simulink model "Dual_Electric_Plant"  (R2021a)
settings: Solver=VariableStepAuto  StartTime=0.0  StopTime=60  RelTol=1e-3  AbsTol=1e-3
InitFcn:
  | Model_Parameters;
undefined symbols (not defined in the file or in its folder): Battery, Electric_Motor, Fuel_Cell
libraries: fl_lib x18, ee_lib x9, nesl_utility x6
settings Model: Creator=jsagardu  LastModifiedBy=LENOVO
settings SolverCC: AutoScaleAbsTol=off  AlgebraicLoopSolver=TrustRegion
settings DebuggingCC: SymbolicDimsDataTypeCodeGenerationDiagnostic=none  SFMachineParentedDataDiag=warning
settings SFSimCC: CustomCodeUndefinedFunction=UseInterfaceOnly
settings SimscapeCC: SimscapeLogType=local  SimscapeLogOpenViewer=on  SimscapeLogLimitData=off  SimscapeLogDataHistory=10000

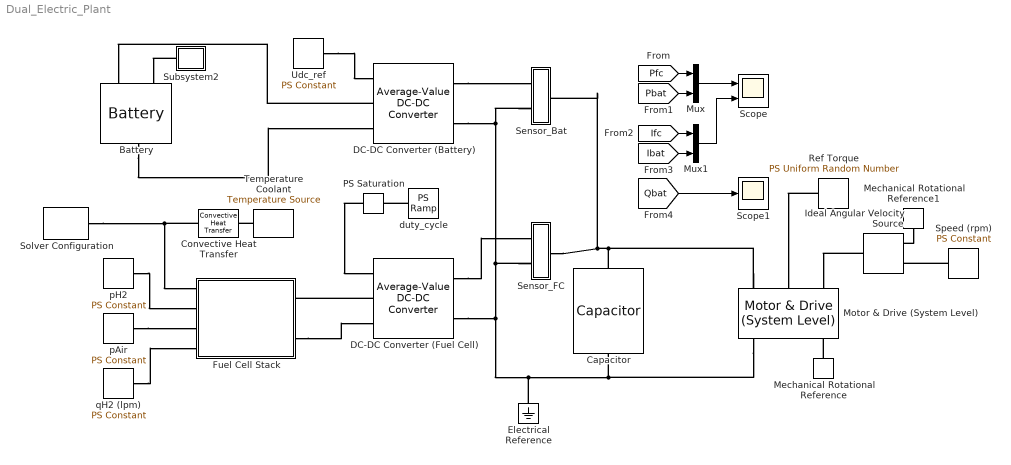
== system Dual_Electric_Plant ==
  Battery : ee_lib/Sources/Battery  Vnom=Battery.Unom V  prm_dir=1  R1_dis=2 Ohm  R1_ch=2 Ohm  R1=Battery.Resistance Ohm  prm_AH=2  AH=Battery.Qnom hr*A  V1=Battery.U1 V  AH1=Battery.Q1 hr*A  prm_R2=1  R2=2000 Ohm  prm_dyn=1  Rp1=0.005 Ohm  tau1=30 s  Rp2=0.005 Ohm  tau2=30 s  Rp3=0.005 Ohm  tau3=30 s  Rp4=0.005 Ohm  tau4=30 s  Rp5=0.005 Ohm  tau5=30 s  prm_fade=1  N_fade=100  AH_fade=45 hr*A  R1_fade=2.02 Ohm  R1_ch_fade=2.02 Ohm  V1_fade=10.35 V  prm_age=1  prm_age_OCV=1  OCV_age=0.9  SOC_age=60  Tmeas_age=298.15 K  delta_time_age_vec=[0] d  temperature_age_vec=[273] K  OCV_scaling_age=2.2134e6  OCV_offset_age=1.632e6  temp_exp_age=0.515833569 V  t_exp_age=0.75  i_specify=off  i_priority=None  i=0 A  i_nominal_specify=off  i_nominal_unit=A  i_nominal_value=1  v_specify=on  v_priority=High  v=Battery.Uinit V  v_nominal_specify=off  v_nominal_unit=V  v_nominal_value=1  charge_specify=on  charge_priority=High  charge=Battery.Qnom hr*A  charge_nominal_specify=off  charge_nominal_unit=hr*A  charge_nominal_value=1  num_cycles_specify=off  num_cycles_priority=High  num_cycles=0  num_cycles_nominal_specify=off  num_cycles_nominal_unit=1  num_cycles_nominal_value=1  thermal_mass=30000 J/K  Tmeas=298.15 K  Vnom_T2=12 V  R1_T2=2.2 Ohm  R1_T2_dis=2.2 Ohm  R1_T2_ch=2.2 Ohm  V1_T2=11.4 V  R2_T2=2200 Ohm  Rp1_T2=0.005 Ohm  tau1_T2=30 s  Rp2_T2=0.005 Ohm  tau2_T2=30 s  Rp3_T2=0.005 Ohm  tau3_T2=30 s  Rp4_T2=0.005 Ohm  tau4_T2=30 s  Rp5_T2=0.005 Ohm  tau5_T2=30 s  Tmeas2=273.15 K  temperature_specify=off  temperature_priority=High  temperature=298.15 K  temperature_nominal_specify=off  temperature_nominal_unit=K  temperature_nominal_value=1
      settings: LogSimulationData=on  InternalSimscapePortConfiguration="{\"Bottom\":[],\"Left\":[{\"id\":\"p\",\"label\":\"+\",\"type\":\"foundation.electrical.electrical\"},{\"id\":\"q\",\"label\":\"q\",\"type\":\"output\"}],\"Right\":[{\"id\":\"n\",\"label\":\"-\",\"type\":\"foundation.electrical.electrical\"}],\"Top\":[]}"
  Capacitor : fl_lib/Electrical/Electrical Elements/Capacitor  c=5 mF  r=0.05 Ohm  g=0 1/Ohm  i_specify=off  i_priority=None  i=0 A  i_nominal_specify=off  i_nominal_unit=A  i_nominal_value=1  v_specify=off  v_priority=None  v=0 V  v_nominal_specify=off  v_nominal_unit=V  v_nominal_value=1  vc_specify=on  vc_priority=High  vc=500 V  vc_nominal_specify=off  vc_nominal_unit=V  vc_nominal_value=1
  Convective Heat Transfer : fl_lib/Thermal/Thermal Elements/Convective Heat Transfer  area=300 cm^2  heat_tr_coeff=75 W/(m^2 * K)  T_specify=off  T_priority=None  T=0 K  T_nominal_specify=off  T_nominal_unit=K  T_nominal_value=1  Q_specify=off  Q_priority=None  Q=0 W  Q_nominal_specify=off  Q_nominal_unit=W  Q_nominal_value=1
  DC-DC Converter (Battery) : ee_lib/Semiconductors & Converters/Converters/Average-Value DC-DC Converter  control_option=ee.enum.converters.controlinput.voltage  converter_type=ee.enum.converters.dcdctype.boost  efficiency_option=ee.enum.converters.efficiency.constant  efficiency_fixed=100  i_vec=[0, 2, 5] A  efficiency_vec=[90, 95, 98]
      settings: SourceProductBaseCode=PS  LogSimulationData=on  InternalSimscapePortConfiguration="{\"Bottom\":[],\"Left\":[{\"id\":\"Vref\",\"label\":\"Vref\",\"type\":\"input\"},{\"id\":\"p1\",\"label\":\"1+\",\"type\":\"foundation.electrical.electrical\"},{\"id\":\"n1\",\"label\":\"1-\",\"type\":\"foundation.electrical.electrical\"}],\"Right\":[{\"id\":\"p2\",\"label\":\"2+\",\"type\":\"foundation.electrical.electrical\"},{\"id\":\"n2\",\"label\":\"2-\",\"type\":\"foundation.electrical.electrical\"}],\"Top\":[]}"
  DC-DC Converter (Fuel Cell) : ee_lib/Semiconductors & Converters/Converters/Average-Value DC-DC Converter  control_option=ee.enum.converters.controlinput.dutycycle  converter_type=ee.enum.converters.dcdctype.boost  efficiency_option=ee.enum.converters.efficiency.constant  efficiency_fixed=100  i_vec=[0, 2, 5] A  efficiency_vec=[90, 95, 98]
      settings: SourceProductBaseCode=PS  LogSimulationData=on  InternalSimscapePortConfiguration="{\"Bottom\":[],\"Left\":[{\"id\":\"DutyCycle\",\"label\":\"DutyCycle\",\"type\":\"input\"},{\"id\":\"p1\",\"label\":\"1+\",\"type\":\"foundation.electrical.electrical\"},{\"id\":\"n1\",\"label\":\"1-\",\"type\":\"foundation.electrical.electrical\"}],\"Right\":[{\"id\":\"p2\",\"label\":\"2+\",\"type\":\"foundation.electrical.electrical\"},{\"id\":\"n2\",\"label\":\"2-\",\"type\":\"foundation.electrical.electrical\"}],\"Top\":[]}"
  Electrical Reference : fl_lib/Electrical/Electrical Elements/Electrical Reference
  Fuel Cell Stack : Subsystem
  Ideal Angular Velocity Source : fl_lib/Mechanical/Mechanical Sources/Ideal Angular Velocity Source
  Mechanical Rotational Reference : fl_lib/Mechanical/Rotational Elements/Mechanical Rotational Reference
  Mechanical Rotational Reference1 : fl_lib/Mechanical/Rotational Elements/Mechanical Rotational Reference
  Motor & Drive (System Level) : ee_lib/Electromechanical/Motor & Drive (System Level)  torque_speed_param=ee.enum.electromech.envelope.torque_power  overtorque_param=ee.enum.electromech.overtorque.no  T_t=[.09, .08, .07, 0] N*m  T_t_intermittent=[.36, .32, .28, 0] N*m  w_t=[0, 3750, 7500, 8000] rpm  torque_max=Electric_Motor.Torque N*m  power_max=Electric_Motor.Power kW  torque_max_intermittent=0.4 N*m  power_max_intermittent=120 W  time_overtorque=30 s  time_recover=60 s  Tc=0.02 s  losses_param=1  eff=100  w_eff=3750 rpm  T_eff=0.08 N*m  Piron=0 W  Pbase=0 W  w_eff_vec=[-8000, -4000, 0, 4000, 8000] rpm  T_eff_vec=[0, .03, .06, .09] N*m  v_eff_vec=[100, 250, 400] V  losses_mat=[1.49, 1.67, 2.21, 3.1; .42, .69, 1.14, 2.03; .06, .24, .78, 1.68; .42, .69, 1.14, 2.03; 1.49, 1.67, 2.21, 3.1] W  efficiency_mat=[95, 95, 95, 95; 95, 95, 95, 95; 95, 95, 95, 95; 95, 95, 95, 95; 95, 95, 95, 95]  losses_mat_3D=ones(5, 4, 3) W  efficiency_mat_3D=95 * ones(5, 4, 3)  Res=0 Ohm  J=5e-6 kg*m^2  lam=1e-5 N*m/(rad/s)  speed0=0 rpm  faulted_specify=off  faulted_priority=None  faulted=0  faulted_nominal_specify=off  faulted_nominal_unit=1  faulted_nominal_value=1  torqueLimitContinuous_specify=off  torqueLimitContinuous_priority=None  torqueLimitContinuous=0 N*m  torqueLimitContinuous_nominal_specify=off  torqueLimitContinuous_nominal_unit=N*m  torqueLimitContinuous_nominal_value=1  alpha=3.93e-3 1/K  Tmeas=25 degC  Tmeas2=125 degC  losses_mat_T2=[1.49, 1.74, 2.49, 3.74; .42, .67, 1.42, 2.67; .06, .31, 1.06, 2.31; .42, .67, 1.42, 2.67; 1.49, 1.74, 2.49, 3.74] W  efficiency_mat_T2=[95, 95, 95, 95; 95, 95, 95, 95; 95, 95, 95, 95; 95, 95, 95, 95; 95, 95, 95, 95]  losses_mat_3D_T2=ones(5, 4, 3) W  efficiency_mat_3D_T2=95 * ones(5, 4, 3)  thermal_mass=100 J/K  initial_temperature=25 degC  fault_condition=1  fault_threshold=0.5
      settings: SourceProductBaseCode=PS
  Mux : Mux  Inputs=2
  Mux1 : Mux  Inputs=2
  PS Saturation : fl_lib/Physical Signals/Nonlinear Operators/PS Saturation  upper_limit=0.95  lower_limit=0.15
      settings: SourceProductBaseCode=SS
  Ref Torque : fl_lib/Physical Signals/Sources/PS Uniform Random Number  minimum=-Electric_Motor.TorqueMin  maximum=Electric_Motor.TorqueMax  initial_seed=0  sample_time=5 s
      settings: SourceProductBaseCode=SS  InternalSimscapePortConfiguration="{\"Bottom\":[],\"Left\":[],\"Right\":[{\"id\":\"Y\",\"label\":\"Y\",\"type\":\"output\"}],\"Top\":[]}"
  Scope : Scope  NumInputPorts=2
  Scope1 : Scope
  Sensor_Bat : Subsystem
  Sensor_FC : Subsystem
  Solver Configuration : nesl_utility/Solver Configuration  PhysicalDomain=network_engine_domain  SubClassName=solver  LeftPortType=input  RightPortType=generic  Tones=[]  Harmonics=[]  SimulateNoise=off  Profile=off  UseLocalSampling=off  EnableSwitchedLinearOptims=on  FrequencyDomain=off  UseCCode=off  RelTol=0.001  AbsTol=1e-06  MinStep=1e-09  ToWorkspace=off  RevertToSquareIcSolve=off  NumHomotopyIterations=100  PhasorMode=off  PhasorModeNumHarmonics=1  DoDC=off  ResidualTolerance=1e-09  UseLocalSolver=off  LocalSolverChoice=NE_BACKWARD_EULER_ADVANCER  LocalSolverSampleTime=0.001  DoFixedCost=off  MaxNonlinIter=3  MaxModeIter=2  ComputeImpulses=off  ImpulseIterations=2  LinearAlgebra=auto  EquationFormulation=NE_TIME_EF  DelaysMemoryBudget=1024  AutomaticFiltering=on  FilteringTimeConstant=0.001  PartitionStorageMethod=AS_NEEDED  PartitionMemoryBudget=1024  PartitionMethod=ROBUST
      settings: SourceProductBaseCode=PW,SS
  Speed (rpm) : fl_lib/Physical Signals/Sources/PS Constant  constant=1500 rpm
  Subsystem2 : Subsystem
  Temperature Coolant : fl_lib/Thermal/Thermal Sources/Temperature Source  temperature=293.15 K
  Udc_ref : fl_lib/Physical Signals/Sources/PS Constant  constant=480
  duty_cycle : fl_lib/Physical Signals/Sources/PS Ramp  slope=-0.8/60 1/s  start_time=0 s  initial_output=0.95
      settings: SourceProductBaseCode=SS
  pAir : fl_lib/Physical Signals/Sources/PS Constant  constant=1 bar
  pH2 : fl_lib/Physical Signals/Sources/PS Constant  constant=5.0 bar
  qH2 (lpm) : fl_lib/Physical Signals/Sources/PS Constant  constant=80 lpm
  wires:
  [Pbat] -> Mux/2
  [Pfc] -> Mux/1
  Mux/1 -> Scope/1
  Mux1/1 -> Scope/2
  [Ifc] -> Mux1/1
  [Ibat] -> Mux1/2
  [Qbat] -> Scope1/1
  connections:
  DC-DC Converter (Battery)/RConn2 -- Sensor_Bat/LConn2 -- Electrical Reference/LConn1 -- Motor & Drive (System Level)/RConn1 -- Capacitor/RConn1 -- DC-DC Converter (Fuel Cell)/RConn2 -- Sensor_FC/LConn2
  Temperature Coolant/LConn1 -- Convective Heat Transfer/RConn1
  Battery/RConn1 -- DC-DC Converter (Battery)/LConn3
  DC-DC Converter (Battery)/LConn2 -- Battery/LConn1
  Udc_ref/RConn1 -- DC-DC Converter (Battery)/LConn1
  duty_cycle/RConn1 -- PS Saturation/LConn1
  Convective Heat Transfer/LConn1 -- Fuel Cell Stack/LConn1 -- Solver Configuration/RConn1
  DC-DC Converter (Fuel Cell)/LConn2 -- Fuel Cell Stack/RConn1
  pH2/RConn1 -- Fuel Cell Stack/LConn2
  pAir/RConn1 -- Fuel Cell Stack/LConn3
  Fuel Cell Stack/RConn2 -- DC-DC Converter (Fuel Cell)/LConn3
  qH2 (lpm)/RConn1 -- Fuel Cell Stack/LConn4
  PS Saturation/RConn1 -- DC-DC Converter (Fuel Cell)/LConn1
  Capacitor/LConn1 -- Motor & Drive (System Level)/LConn1 -- Sensor_Bat/RConn1 -- Sensor_FC/RConn1
  DC-DC Converter (Battery)/RConn1 -- Sensor_Bat/LConn1
  DC-DC Converter (Fuel Cell)/RConn1 -- Sensor_FC/LConn1
  Subsystem2/LConn1 -- Battery/LConn2
  Mechanical Rotational Reference/LConn1 -- Motor & Drive (System Level)/RConn3
  Ideal Angular Velocity Source/LConn1 -- Motor & Drive (System Level)/LConn3
  Mechanical Rotational Reference1/LConn1 -- Ideal Angular Velocity Source/RConn2
  Ref Torque/RConn1 -- Motor & Drive (System Level)/LConn2
  Speed (rpm)/RConn1 -- Ideal Angular Velocity Source/RConn1

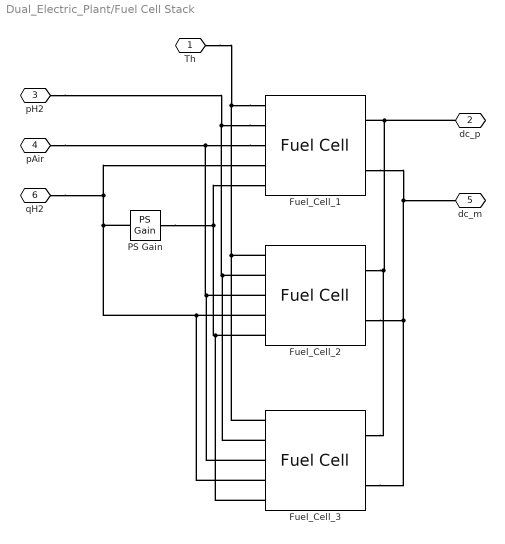
== system Dual_Electric_Plant/Fuel Cell Stack ==
  Fuel_Cell_1 : ee_lib/Sources/Fuel Cell  model_fidelity=ee.enum.fuelcell.fidelity.detailed  Eoc=Fuel_Cell.OC_Voltage V  A=Fuel_Cell.Tafel_Slope V  ri=Fuel_Cell.Resistance Ohm  i0=Fuel_Cell.Exchange_Current A  N_cell=65  number_unit=10  dyn=ee.enum.include.no  i_lim=Fuel_Cell.Collapse_Current A  Tnom=293.15 K  thermal_mass=30000 J/K  pH2_nom=Fuel_Cell.pH2_nom Pa  pO2_nom=Fuel_Cell.pAir_nom Pa  xH2=99  xO2=21  xW=1  Rd=0.005 Ohm  tau=10 s  iFC_specify=off  iFC_priority=None  iFC=0 A  iFC_nominal_specify=off  iFC_nominal_unit=A  iFC_nominal_value=1  vFC_specify=off  vFC_priority=None  vFC=0 V  vFC_nominal_specify=off  vFC_nominal_unit=V  vFC_nominal_value=1  temperature_specify=off  temperature_priority=High  temperature=293 K  temperature_nominal_specify=off  temperature_nominal_unit=K  temperature_nominal_value=1
      settings: SourceProductBaseCode=PS  LogSimulationData=on  InternalSimscapePortConfiguration="{\"Bottom\":[],\"Left\":[{\"id\":\"H\",\"label\":\"H\",\"type\":\"foundation.thermal.thermal\"},{\"id\":\"pfuel\",\"label\":\"pfuel\",\"type\":\"input\"},{\"id\":\"pair\",\"label\":\"pair\",\"type\":\"input\"},{\"id\":\"qfuel\",\"label\":\"qfuel\",\"type\":\"input\"},{\"id\":\"qair\",\"label\":\"qair\",\"type\":\"input\"}],\"Right\":[{\"id\":\"p\",\"label\":\"+\",\"type\":\"foundation.electrical.electrical\"},{\"id\":\"n\",\"label\":\"-\",\"type\":\"foundation.electrical.electrical\"}],\"Top\":[]}"
  Fuel_Cell_2 : ee_lib/Sources/Fuel Cell  model_fidelity=ee.enum.fuelcell.fidelity.detailed  Eoc=Fuel_Cell.OC_Voltage V  A=Fuel_Cell.Tafel_Slope V  ri=Fuel_Cell.Resistance Ohm  i0=Fuel_Cell.Exchange_Current A  N_cell=65  number_unit=10  dyn=ee.enum.include.no  i_lim=Fuel_Cell.Collapse_Current A  Tnom=293.15 K  thermal_mass=30000 J/K  pH2_nom=Fuel_Cell.pH2_nom Pa  pO2_nom=Fuel_Cell.pAir_nom Pa  xH2=99  xO2=21  xW=1  Rd=0.005 Ohm  tau=10 s  iFC_specify=off  iFC_priority=None  iFC=0 A  iFC_nominal_specify=off  iFC_nominal_unit=A  iFC_nominal_value=1  vFC_specify=off  vFC_priority=None  vFC=0 V  vFC_nominal_specify=off  vFC_nominal_unit=V  vFC_nominal_value=1  temperature_specify=off  temperature_priority=High  temperature=293 K  temperature_nominal_specify=off  temperature_nominal_unit=K  temperature_nominal_value=1
      settings: SourceProductBaseCode=PS  LogSimulationData=on  InternalSimscapePortConfiguration="{\"Bottom\":[],\"Left\":[{\"id\":\"H\",\"label\":\"H\",\"type\":\"foundation.thermal.thermal\"},{\"id\":\"pfuel\",\"label\":\"pfuel\",\"type\":\"input\"},{\"id\":\"pair\",\"label\":\"pair\",\"type\":\"input\"},{\"id\":\"qfuel\",\"label\":\"qfuel\",\"type\":\"input\"},{\"id\":\"qair\",\"label\":\"qair\",\"type\":\"input\"}],\"Right\":[{\"id\":\"p\",\"label\":\"+\",\"type\":\"foundation.electrical.electrical\"},{\"id\":\"n\",\"label\":\"-\",\"type\":\"foundation.electrical.electrical\"}],\"Top\":[]}"
  Fuel_Cell_3 : ee_lib/Sources/Fuel Cell  model_fidelity=ee.enum.fuelcell.fidelity.detailed  Eoc=Fuel_Cell.OC_Voltage V  A=Fuel_Cell.Tafel_Slope V  ri=Fuel_Cell.Resistance Ohm  i0=Fuel_Cell.Exchange_Current A  N_cell=65  number_unit=10  dyn=ee.enum.include.no  i_lim=Fuel_Cell.Collapse_Current A  Tnom=293.15 K  thermal_mass=30000 J/K  pH2_nom=Fuel_Cell.pH2_nom Pa  pO2_nom=Fuel_Cell.pAir_nom Pa  xH2=99  xO2=21  xW=1  Rd=0.005 Ohm  tau=10 s  iFC_specify=off  iFC_priority=None  iFC=0 A  iFC_nominal_specify=off  iFC_nominal_unit=A  iFC_nominal_value=1  vFC_specify=off  vFC_priority=None  vFC=0 V  vFC_nominal_specify=off  vFC_nominal_unit=V  vFC_nominal_value=1  temperature_specify=off  temperature_priority=High  temperature=293 K  temperature_nominal_specify=off  temperature_nominal_unit=K  temperature_nominal_value=1
      settings: SourceProductBaseCode=PS  LogSimulationData=on  InternalSimscapePortConfiguration="{\"Bottom\":[],\"Left\":[{\"id\":\"H\",\"label\":\"H\",\"type\":\"foundation.thermal.thermal\"},{\"id\":\"pfuel\",\"label\":\"pfuel\",\"type\":\"input\"},{\"id\":\"pair\",\"label\":\"pair\",\"type\":\"input\"},{\"id\":\"qfuel\",\"label\":\"qfuel\",\"type\":\"input\"},{\"id\":\"qair\",\"label\":\"qair\",\"type\":\"input\"}],\"Right\":[{\"id\":\"p\",\"label\":\"+\",\"type\":\"foundation.electrical.electrical\"},{\"id\":\"n\",\"label\":\"-\",\"type\":\"foundation.electrical.electrical\"}],\"Top\":[]}"
  PS Gain : fl_lib/Physical Signals/Functions/PS Gain  gain=3
  Th : PMIOPort  Side=Left
  dc_p : PMIOPort  Port=2  Side=Right
  pH2 : PMIOPort  Port=3  Side=Left
  pAir : PMIOPort  Port=4  Side=Left
  dc_m : PMIOPort  Port=5  Side=Right
  qH2 : PMIOPort  Port=6  Side=Left
  connections:
  Fuel_Cell_1/RConn2 -- Fuel_Cell_3/RConn2 -- Fuel_Cell_2/RConn2 -- dc_m/RConn1
  Fuel_Cell_1/RConn1 -- dc_p/RConn1 -- Fuel_Cell_3/RConn1 -- Fuel_Cell_2/RConn1
  Fuel_Cell_1/LConn2 -- pH2/RConn1 -- Fuel_Cell_3/LConn2 -- Fuel_Cell_2/LConn2
  PS Gain/RConn1 -- Fuel_Cell_3/LConn5 -- Fuel_Cell_2/LConn5 -- Fuel_Cell_1/LConn5
  Fuel_Cell_3/LConn4 -- Fuel_Cell_2/LConn4 -- PS Gain/LConn1 -- qH2/RConn1 -- Fuel_Cell_1/LConn4
  Fuel_Cell_1/LConn3 -- pAir/RConn1 -- Fuel_Cell_3/LConn3 -- Fuel_Cell_2/LConn3
  Fuel_Cell_1/LConn1 -- Th/RConn1 -- Fuel_Cell_2/LConn1 -- Fuel_Cell_3/LConn1

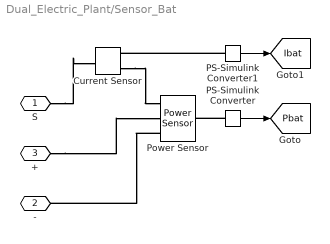
== system Dual_Electric_Plant/Sensor_Bat ==
  Current Sensor : fl_lib/Electrical/Electrical Sensors/Current Sensor
  PS-Simulink Converter : nesl_utility/PS-Simulink Converter  PhysicalDomain=network_engine_domain  SubClassName=ps_output  LeftPortType=input  RightPortType=output  PseudoPeriodic=off  Frequencies=[]  Unit=kW  AffineConversion=off
      settings: SourceProductBaseCode=PW,SS
  PS-Simulink Converter1 : nesl_utility/PS-Simulink Converter  PhysicalDomain=network_engine_domain  SubClassName=ps_output  LeftPortType=input  RightPortType=output  PseudoPeriodic=off  Frequencies=[]  Unit=A  AffineConversion=off
      settings: SourceProductBaseCode=PW,SS
  Power Sensor : ee_lib/Sensors & Transducers/Power Sensor  measurement_type=1  averaging_period=1e-4 s
      settings: SourceProductBaseCode=PS
  S : PMIOPort  Side=Left
  - : PMIOPort  Port=2  Side=Left
  + : PMIOPort  Port=3  Side=Right
  tag scope: Ibat=global, Pbat=global
  wires:
  PS-Simulink Converter/1 -> [Pbat]
  PS-Simulink Converter1/1 -> [Ibat]
  connections:
  +/RConn1 -- Power Sensor/LConn2
  Power Sensor/LConn3 -- -/RConn1
  PS-Simulink Converter/LConn1 -- Power Sensor/RConn1
  Current Sensor/RConn2 -- Power Sensor/LConn1
  S/RConn1 -- Current Sensor/LConn1
  PS-Simulink Converter1/LConn1 -- Current Sensor/RConn1

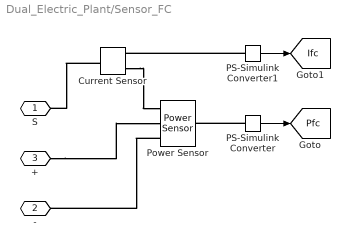
== system Dual_Electric_Plant/Sensor_FC ==
  Current Sensor : fl_lib/Electrical/Electrical Sensors/Current Sensor
  PS-Simulink Converter : nesl_utility/PS-Simulink Converter  PhysicalDomain=network_engine_domain  SubClassName=ps_output  LeftPortType=input  RightPortType=output  PseudoPeriodic=off  Frequencies=[]  Unit=kW  AffineConversion=off
      settings: SourceProductBaseCode=PW,SS
  PS-Simulink Converter1 : nesl_utility/PS-Simulink Converter  PhysicalDomain=network_engine_domain  SubClassName=ps_output  LeftPortType=input  RightPortType=output  PseudoPeriodic=off  Frequencies=[]  Unit=A  AffineConversion=off
      settings: SourceProductBaseCode=PW,SS
  Power Sensor : ee_lib/Sensors & Transducers/Power Sensor  measurement_type=1  averaging_period=1e-4 s
      settings: SourceProductBaseCode=PS
  S : PMIOPort  Side=Left
  - : PMIOPort  Port=2  Side=Left
  + : PMIOPort  Port=3  Side=Right
  tag scope: Ifc=global, Pfc=global
  wires:
  PS-Simulink Converter/1 -> [Pfc]
  PS-Simulink Converter1/1 -> [Ifc]
  connections:
  +/RConn1 -- Power Sensor/LConn2
  Power Sensor/LConn3 -- -/RConn1
  PS-Simulink Converter/LConn1 -- Power Sensor/RConn1
  PS-Simulink Converter1/LConn1 -- Current Sensor/RConn1
  Current Sensor/LConn1 -- S/RConn1
  Current Sensor/RConn2 -- Power Sensor/LConn1

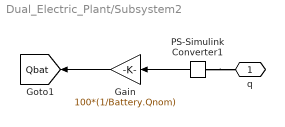
== system Dual_Electric_Plant/Subsystem2 ==
  Gain : Gain  Gain=100*(1/Battery.Qnom)
  PS-Simulink Converter1 : nesl_utility/PS-Simulink Converter  PhysicalDomain=network_engine_domain  SubClassName=ps_output  LeftPortType=input  RightPortType=output  PseudoPeriodic=off  Frequencies=[]  Unit=A*hr  AffineConversion=off
      settings: SourceProductBaseCode=PW,SS
  q : PMIOPort  Side=Left
  tag scope: Qbat=global
  wires:
  PS-Simulink Converter1/1 -> Gain/1
  Gain/1 -> [Qbat]
  connections:
  PS-Simulink Converter1/LConn1 -- q/RConn1
